simulink model "controlPID"  (R2018a)
settings: Solver=VariableStepAuto  StartTime=0.0  StopTime=10  RelTol=1e-3
libraries: simulink x1
settings Model: Creator=robotica  LastModifiedBy=JMONTIELG
settings CodeAppCC: StateflowObjectComments=on

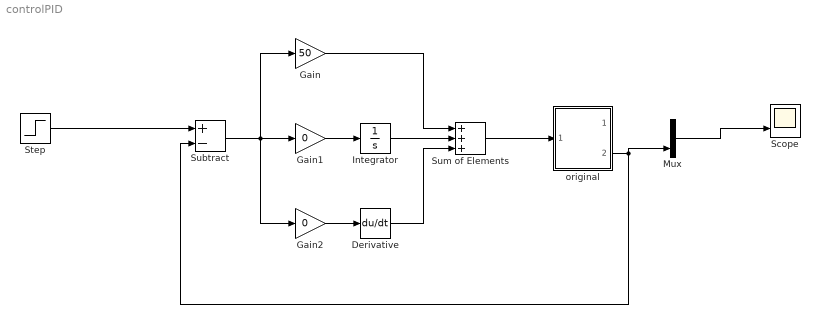
== system controlPID ==
  Derivative : Derivative  CoefficientInTFapproximation=1
  Gain : Gain  Gain=50
  Gain1 : Gain  Gain=0
  Gain2 : Gain  Gain=0
  Integrator : Integrator
  Mux : Mux  Inputs=2
  Scope : Scope  NumInputPorts=2
  Step : Step  SampleTime=1
  Subtract : Sum  Inputs=+-
  Sum of Elements : Sum  Inputs=+++
  original : Subsystem
  wires:
  original/2(clean) -> Mux/2, Subtract/2
  Gain/1 -> Sum of Elements/1
  Integrator/1 -> Sum of Elements/2
  Sum of Elements/1 -> original/1(signal)
  Derivative/1 -> Sum of Elements/3
  Gain1/1 -> Integrator/1
  Step/1 -> Subtract/1
  Subtract/1 -> Gain2/1, Gain1/1, Gain/1
  Mux/1 -> Scope/2
  Gain2/1 -> Derivative/1

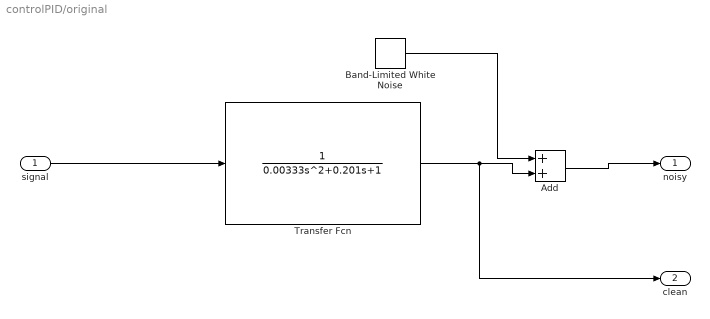
== system controlPID/original ==
  signal : Inport
  Add : Sum
  Band-Limited White Noise : simulink/Sources/Band-Limited White Noise  Cov=[0.0000001]  Ts=0.001  seed=[23341]
  Transfer Fcn : TransferFcn  Denominator=[0.00333 0.201 1]
  noisy : Outport
  clean : Outport  Port=2
  wires:
  Transfer Fcn/1 -> clean/1, Add/2
  Band-Limited White Noise/1 -> Add/1
  Add/1 -> noisy/1
  signal/1 -> Transfer Fcn/1
